simulink model "estimator"  (R2015b)
settings: Solver=VariableStepAuto  StartTime=0.0  StopTime=20.0  RelTol=1e-3
values from neighbouring files (symbols this model uses):
  A = [zeros(2) eye(2); -inv(M)*kappa -inv(M)*beta]    [Lab3_Solution.m]    (also in lab4.m = [0 0 1 0; 0 0 0 1; 0 (mp^2 * l^2 *g)/mu (-c*Jt)/mu (-Y*Jt*l*; lab4_pid_controller.m; lab4_state_feedback_no_estimator.m; lab4_state_feedback_with_estimator.m)
  B = [0; 0; inv(M)*S]    [Lab3_Solution.m]    (also in lab4.m = [0; 0; Jt/mu; (l*mp)/mu]; lab4_pid_controller.m; lab4_state_feedback_no_estimator.m; lab4_state_feedback_with_estimator.m)
  C = [1 0 0 0; 0 1 0 0]    [Lab3_Solution.m]    (also in PendulumTutorial.m = zpk(z,p,k); lab4.m; lab4_pid_controller.m = eye(4); lab4_state_feedback_no_estimator.m = eye(4))
  D = [0; 0]    [Lab3_Solution.m]    (also in lab4.m; lab4_pid_controller.m = [0; 0; 0; 0]; lab4_state_feedback_no_estimator.m = [0; 0; 0; 0]; lab4_state_feedback_with_estimator.m)
  K = 20    [PendulumTutorial.m]    (also in lab4_state_feedback_no_estimator.m = place(A,B,p); lab4_state_feedback_with_estimator.m = place(A,B,p))
  kr = -1/(C*inv(A-B*K)*B)    [lab4_state_feedback_no_estimator.m]    (also in lab4_state_feedback_with_estimator.m)
  L = place(A',C',[-1 -1.1 -1.01 -1.001])'    [lab4_state_feedback_with_estimator.m]
settings Model: Creator=lukasgemar  LastModifiedBy=Lukas Gemar

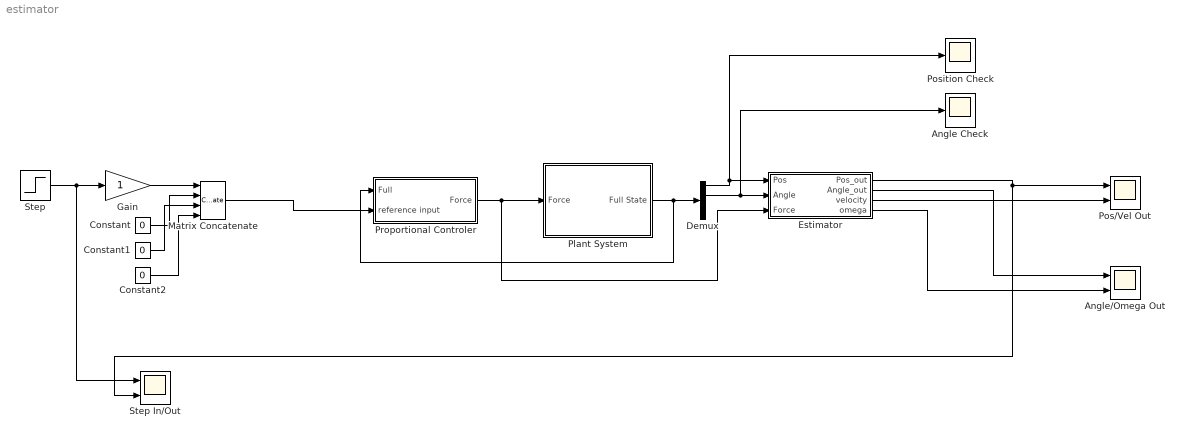
== system estimator ==
  Angle Check : Scope
  Angle/Omega Out : Scope  NumInputPorts=2
  Constant : Constant  Value=0
  Constant1 : Constant  Value=0
  Constant2 : Constant  Value=0
  Demux : Demux
  Estimator : Subsystem
  Gain : Gain
  Matrix Concatenate : Concatenate  NumInputs=4  Mode=Multidimensional array
  Plant System : Subsystem
  Pos/Vel Out : Scope  NumInputPorts=2
  Position Check : Scope
  Proportional Controler : Subsystem
  Step : Step  SampleTime=0
  "Step In/Out " : Scope  NumInputPorts=2
  wires:
  Step/1 -> Gain/1, "Step In/Out "/1
  Proportional Controler/1(Force) -> Estimator/3(Force), Plant System/1(Force)
  Estimator/1(Pos_out) -> "Step In/Out "/2, Pos/Vel Out/1
  Estimator/2("Angle_out ") -> Angle/Omega Out/1
  Estimator/3("velocity ") -> Pos/Vel Out/2
  Estimator/4(omega) -> Angle/Omega Out/2
  Plant System/1(Full State) -> Proportional Controler/1(Full), Demux/1
  Gain/1 -> Matrix Concatenate/1
  Constant/1 -> Matrix Concatenate/2
  Constant1/1 -> Matrix Concatenate/3
  Constant2/1 -> Matrix Concatenate/4
  Matrix Concatenate/1 -> Proportional Controler/2(reference input)
  Demux/1 -> Estimator/1(Pos), Position Check/1
  Demux/2 -> Angle Check/1, Estimator/2(Angle)

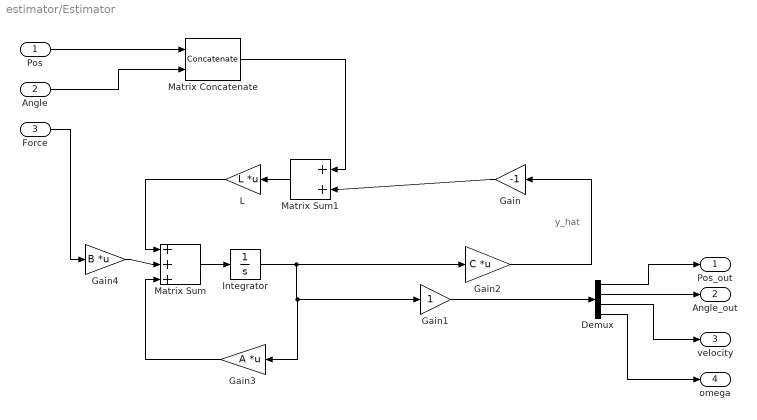
== system estimator/Estimator ==
  note: y_hat
  Pos : Inport
  Angle : Inport  Port=2
  Force : Inport  Port=3
  Demux : Demux
  Gain : Gain  Gain=-1
  Gain1 : Gain
  Gain2 : Gain  Gain=C  Multiplication=Matrix(K*u)
  Gain3 : Gain  Gain=A  Multiplication=Matrix(K*u)
  Gain4 : Gain  Gain=B  Multiplication=Matrix(K*u)
  Integrator : Integrator
  L : Gain  Gain=L  Multiplication=Matrix(K*u)
  Matrix Concatenate : Concatenate  Mode=Multidimensional array
  Matrix Sum : Sum  Inputs=+++|  InputSameDT=on
  Matrix Sum1 : Sum  Inputs=++|
  Pos_out : Outport
  "Angle_out " : Outport  Port=2
  "velocity " : Outport  Port=3
  omega : Outport  Port=4
  wires:
  Pos/1 -> Matrix Concatenate/1
  Angle/1 -> Matrix Concatenate/2
  Gain/1 -> Matrix Sum1/2
  Gain2/1 -> Gain/1
  Integrator/1 -> Gain3/1, Gain1/1, Gain2/1
  Demux/1 -> Pos_out/1
  Demux/2 -> "Angle_out "/1
  Demux/3 -> "velocity "/1
  Demux/4 -> omega/1
  Force/1 -> Gain4/1
  Gain4/1 -> Matrix Sum/2
  L/1 -> Matrix Sum/1
  Matrix Sum/1 -> Integrator/1
  Gain3/1 -> Matrix Sum/3
  Matrix Sum1/1 -> L/1
  Matrix Concatenate/1 -> Matrix Sum1/1
  Gain1/1 -> Demux/1

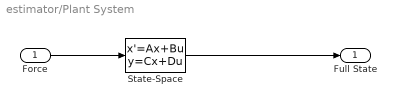
== system estimator/Plant System ==
  Force : Inport
  State-Space : StateSpace  A=A  B=B  C=C  D=D  X0=[0;0;0;0]
  Full State : Outport
  wires:
  Force/1 -> State-Space/1
  State-Space/1 -> Full State/1

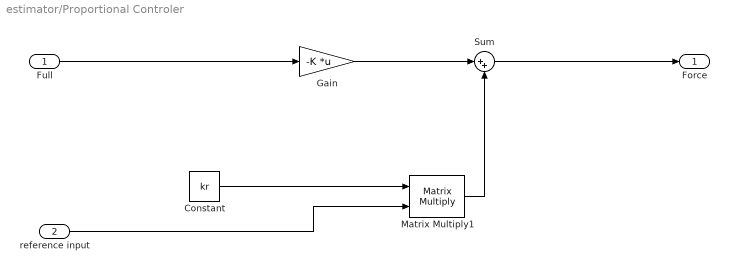
== system estimator/Proportional Controler ==
  Full : Inport
  reference input : Inport  Port=2
  Constant : Constant  Value=kr  VectorParams1D=off
  Gain : Gain  Gain=-K  Multiplication=Matrix(K*u)
  Matrix Multiply1 : Product  Multiplication=Matrix(*)
  Sum : Sum  Inputs=|++
  Force : Outport
  wires:
  Gain/1 -> Sum/1
  Sum/1 -> Force/1
  Matrix Multiply1/1 -> Sum/2
  Constant/1 -> Matrix Multiply1/1
  reference input/1 -> Matrix Multiply1/2
  Full/1 -> Gain/1
